simulink model "ConvertPWMtoAngle"  (R2020b)
settings: Solver=FixedStepDiscrete  StartTime=0.0  StopTime=10.0  FixedStep=4*Ts  RelTol=1e-3
values from neighbouring files (symbols this model uses):
  Angle_T = 0.0 0.001533 0.003066 0.004599 0.006132 0.007665 0.009198 0.010731 0.012264 0.013797 0.01533 0.016863 0.018396 0.019929 0.021462 0.022995 0.024528 0.026061 0.027594 0.029127 0.03066 0.032193 0.033726 0.035259 0.036792 0.038325 0.039858 0.041391 0.042924 0.044457 0.04599 0.047523 0.049056 0.050589 0.052122 0.053655 0.055188 0.056721 0.058254 0.059787 0.06132 0.062853 0.064386 0.065919 0.067452 0.06    [PWMtoAngle.sldd]
  p = 4.0    [CalcSpeednDir.sldd]    (also in MotorControl.sldd)
settings Model: DataDictionary=PWMtoAngle.sldd  Creator=nikotosi  LastModifiedBy=unix
settings OptimizationCC: DefaultParameterBehavior=Inlined  EnhancedBackFolding=on  PassReuseOutputArgsAs=Individual arguments  ZeroExternalMemoryAtStartup=off  ZeroInternalMemoryAtStartup=off  OptimizeBlockOrder=speed  DifferentSizesBufferReuse=on  OptimizationCustomize=off  EfficientTunableParamExpr=on
settings DebuggingCC: ParameterTunabilityLossMsg=error
settings SFSimCC: MATLABDynamicMemAlloc=off
settings RTWCC: Description=Embedded Coder  SystemTargetFile=ert.tlc  GenCodeOnly=on  TemplateMakefile=ert_default_tmf  GenerateReport=on  IncludeHyperlinkInReport=on  LaunchReport=on  GenerateTraceInfo=on  GenerateTraceReport=on  GenerateTraceReportSl=on  GenerateTraceReportSf=on  GenerateTraceReportEml=on
settings CodeAppCC: ForceParamTrailComments=on  IgnoreCustomStorageClasses=off  OperatorAnnotations=on  SimulinkDataObjDesc=on  SFDataObjDesc=on  InsertBlockDesc=on
settings ERTTargetCC: TargetLangStandard=C99 (ISO)  GenerateSampleERTMain=on  InlinedParameterPlacement=NonHierarchical  ERTCustomFileTemplate=example_file_process.tlc

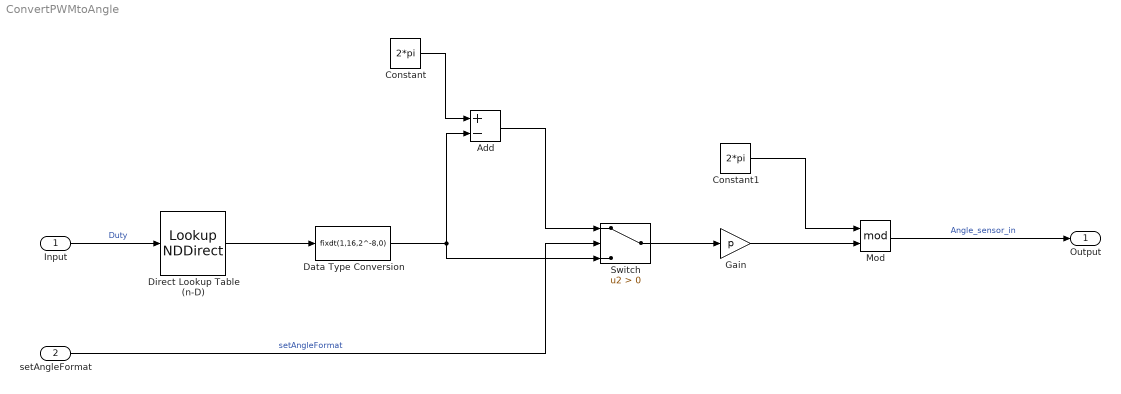
== system ConvertPWMtoAngle ==
  Input : Inport  OutDataTypeStr=uint16
  setAngleFormat : Inport  Port=2  OutDataTypeStr=boolean
  Add : Sum  Inputs=+-
  Constant : Constant  Value=2*pi  OutDataTypeStr=fixdt(1,16,2^-8,0)
  Constant1 : Constant  Value=2*pi  OutDataTypeStr=single
  Data Type Conversion : DataTypeConversion  OutDataTypeStr=fixdt(1,16,2^-8,0)
  Direct Lookup Table (n-D) : LookupNDDirect  NumberOfTableDimensions=1  Table=Angle_T
  Gain : Gain  Gain=p  OutDataTypeStr=single  RndMeth=Simplest
  Mod : Math  Operator=mod  OutputSignalType=real  SaturateOnIntegerOverflow=on
  Switch : Switch  Criteria=u2 > Threshold
  Output : Outport
  wires:
  Input/1 -> Direct Lookup Table (n-D)/1  "Duty"
  Data Type Conversion/1 -> Switch/3, Add/2
  Direct Lookup Table (n-D)/1 -> Data Type Conversion/1
  Constant/1 -> Add/1
  Mod/1 -> Output/1  "Angle_sensor_in"
  setAngleFormat/1 -> Switch/2  "setAngleFormat"
  Add/1 -> Switch/1
  Switch/1 -> Gain/1
  Gain/1 -> Mod/2
  Constant1/1 -> Mod/1
